simulink model "MS_test"  (R2023b)
settings: Solver=VariableStepAuto  StartTime=0.0  StopTime=10.0  RelTol=1e-3
PostLoadFcn:
  | myOutBus= Simulink.Bus;
  | el1=Simulink.BusElement;
  | el1.Name = 'rresult';
  | el1.DataType = 'Bus: rresult';
  | el2=Simulink.BusElement;
  | el2.Name = 'eresult';
  | el2.DataType = 'Bus: eresult';
  | el3 = Simulink.BusElement;
  | el3.Name = 'cresult';
  | el3.DataType = 'Bus: cresult';
  | 
  | eresult = Simulink.Bus;
  | eel1 = Simulink.BusElement;
  | eel1.Name = 'state';
  | eel1.Dimensions = [12 1];
  | eel2 = Simulink.BusElement;
  | eel2.Name = 'P';
  | eel2.Dimensions = [12 12];
  | eel3 = Simulink.BusElement;
  | eel3.Name = 'G';
  | eel3.Dimensions = [12 6];
  | eresult.Elements = [eel1 eel2 eel3];
  | 
  | cresult = Simulink.Bus;
  | cel0 = Simulink.BusElement;
  | cel0.Name = 'input';
  | cel0.Dimensions = [4 1];
  | cresult.Elements = cel0;
  | 
  | rresult = Simulink.Bus;
  | rel0 = Simulink.BusElement;
  | rel0.Name = 'state';
  | rel0.DataType = 'Bus: rstate';
  | rresult.Elements = rel0;
  | 
  | rstate = Simulink.Bus;
  | rsel0 = Simulink.BusElement;
  | rsel0.Name = 'xd';
  | rsel0.Dimensions = [20 1];
  | rsel1 = Simulink.BusElement;
  | rsel1.Name = 'p';
  | rsel1.Dimensions = [3 1];
  | rsel2 = Simulink.BusElement;
  | rsel2.Name = 'v';
  | rsel2.Dimensions = [3 1];
  | rsel3 = Simulink.BusElement;
  | rsel3.Name = 'q';
  | rsel3.Dimensions = [3 1];
  | 
  | rstate.Elements = [rsel0 rsel1 rsel2 rsel3];
  | 
  | myOutBus.Elements = [el1 el2 el3];
values from neighbouring files (symbols this model uses):
  dt = 0.025    [9_26_1.mat]    (also in CONTROLLER_SYSTEM.m = 0.01; Copy_of_drone_model.m = "double")
  x0 = [1;0]    [Copy_of_drone_model.m]
settings Model: Creator=kasek  LastModifiedBy=sekiguchi

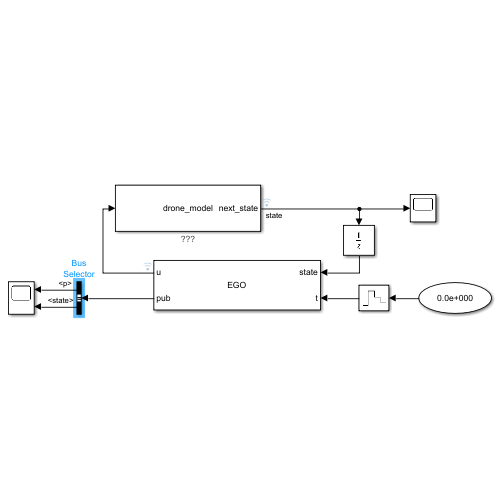
[thumbnail: Simulink's stored preview of the top-level diagram]
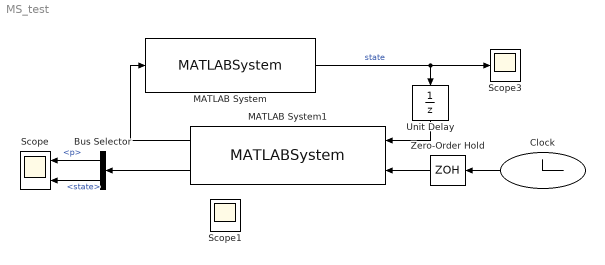
== system MS_test ==
  Bus Selector : BusSelector  OutputSignals=rresult.state.p,eresult.state
  Clock : Clock
  MATLAB System : MATLABSystem  System=drone_model  SimulateUsing=Code generation
      settings: AttributesFormatString=%<A>
      mask Type: drone_model
      mask Display:
      | disp('drone_model');
      | port_label('output',1,'next_state');
  MATLAB System1 : MATLABSystem  System=EGO  SimulateUsing=Code generation
      mask Type: EGO
      mask Display:
      | disp('EGO');
      | port_label('input',1,'state');
      | port_label('input',2,'t');
      | port_label('output',1,'u');
      | port_label('output',2,'pub');
  Scope : Scope  NumInputPorts=2
  Scope3 : Scope
  Unit Delay : UnitDelay  InitialCondition=x0  SampleTime=dt  HasFrameUpgradeWarning=on
  Zero-Order Hold : ZeroOrderHold  SampleTime=dt
  Scope1 : Scope
  wires:
  MATLAB System/1 -> Scope3/1, Unit Delay/1  "state"
  Clock/1 -> Zero-Order Hold/1
  Zero-Order Hold/1 -> MATLAB System1/2
  MATLAB System1/1 -> MATLAB System/1
  Unit Delay/1 -> MATLAB System1/1
  Bus Selector/1 -> Scope/1  "<p>"
  Bus Selector/2 -> Scope/2  "<state>"
  MATLAB System1/2 -> Bus Selector/1
